simulink model "SWC_CGW_type"  (R2021b)
settings: Solver=FixedStepDiscrete  StartTime=0.0  StopTime=10.0  RelTol=1e-3
(part 1 of 3)
settings Model: DataDictionary=APPTypes.sldd  Creator=FVT23010  LastModifiedBy=FVT23118
settings DataIOCC: SaveFormat=StructureWithTime
settings OptimizationCC: DefaultParameterBehavior=Inlined  EnhancedBackFolding=on  PassReuseOutputArgsAs=Individual arguments  ZeroExternalMemoryAtStartup=off  ZeroInternalMemoryAtStartup=off  OptimizeBlockOrder=speed  DifferentSizesBufferReuse=on  OptimizationCustomize=off  EfficientTunableParamExpr=on
settings DebuggingCC: ParameterTunabilityLossMsg=error
settings HardwareCC: ProdBitPerPointer=32  ProdBitPerSizeT=32  ProdBitPerPtrDiffT=32  ProdLargestAtomicInteger=Long  ProdLargestAtomicFloat=Double  ProdWordSize=32  ProdLongLongMode=on  ProdHWDeviceType=ARM Compatible->ARM Cortex-M
settings ModelReferenceCC: ModelReferenceNumInstancesAllowed=Single
settings SFSimCC: MATLABDynamicMemAlloc=off
settings RTWCC: Description=AUTOSAR  SystemTargetFile=autosar.tlc  GenCodeOnly=on  TemplateMakefile=ert_default_tmf  PortableWordSizes=on
settings CodeAppCC: ForceParamTrailComments=on  IgnoreCustomStorageClasses=off  OperatorAnnotations=on  SimulinkDataObjDesc=on  SFDataObjDesc=on  InsertBlockDesc=on
settings STFCustomTargetCC: TargetLangStandard=C99 (ISO)  MultiwordLength=256  ParMdlRefBuildCompliant=on  CompOptLevelCompliant=on  IncludeMdlTerminateFcn=off  CombineOutputUpdateFcns=on  SuppressErrorStatus=on  ERTCustomFileBanners=on  SupportNonFinite=off  SupportComplex=off  SupportContinuousTime=off  SupportNonInlinedSFcns=off  RemoveResetFunc=on  MATLABClassNameForMDSCustomization=Simulink.SoftwareTarget.ERTCustomization  AutosarCompliant=on  GRTInterface=off  UseToolchainInfoCompliant=on  LookupTableObjectStructAxisOrder=2,1,3,4,...  LUTObjectStructOrderEvenSpacing=Size,Table,Breakpoints  SystemTargetFile=autosar.tlc
settings ERTTargetCC: TargetLangStandard=C99 (ISO)  ConcurrentExecutionCompliant=off  IncludeMdlTerminateFcn=off  SuppressErrorStatus=on  SupportNonFinite=off  SupportComplex=off  ModelStepFunctionPrototypeControlCompliant=off  CPPClassGenCompliant=off  AutosarCompliant=on  LookupTableObjectStructAxisOrder=2,1,3,4,...  LUTObjectStructOrderEvenSpacing=Size,Table,Breakpoints  GenerateASAP2=on  InlinedParameterPlacement=NonHierarchical  ERTCustomFileTemplate=example_file_process.tlc  ConvertIfToSwitch=off  SuppressUnreachableDefaultCases=off  BooleanTrueId=true_MatlabRTW  BooleanFalseId=false_MatlabRTW

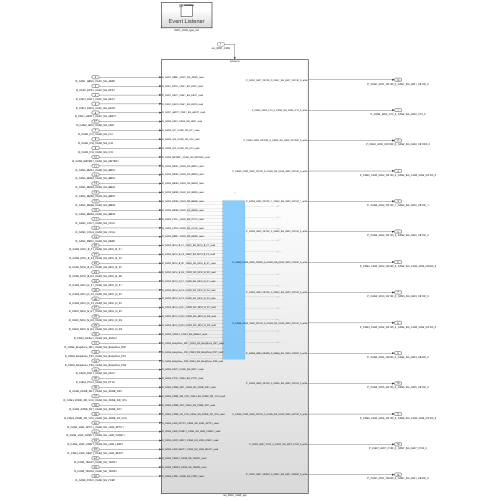
[thumbnail: Simulink's stored preview of the top-level diagram]
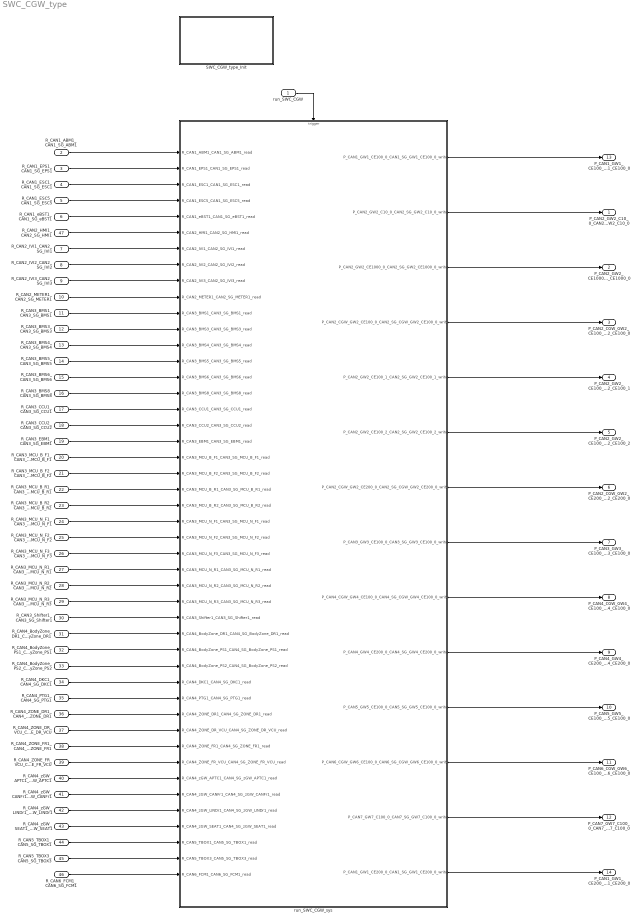
== system SWC_CGW_type ==
  run_SWC_CGW : Inport  OutputFunctionCall=on
  R_CAN1_ABM1_CAN1_SG_ABM1 : Inport  Port=2  OutDataTypeStr=Bus: DT_CAN1_SG_ABM1  PortDimensions=1  BusOutputAsStruct=on
  R_CAN1_EPS1_CAN1_SG_EPS1 : Inport  Port=3  OutDataTypeStr=Bus: DT_CAN1_SG_EPS1  PortDimensions=1  BusOutputAsStruct=on
  R_CAN1_ESC1_CAN1_SG_ESC1 : Inport  Port=4  OutDataTypeStr=Bus: DT_CAN1_SG_ESC1  PortDimensions=1  BusOutputAsStruct=on
  R_CAN1_ESC5_CAN1_SG_ESC5 : Inport  Port=5  OutDataTypeStr=Bus: DT_CAN1_SG_ESC5  PortDimensions=1  BusOutputAsStruct=on
  R_CAN1_eBST1_CAN1_SG_eBST1 : Inport  Port=6  OutDataTypeStr=Bus: DT_CAN1_SG_eBST1  PortDimensions=1  BusOutputAsStruct=on
  R_CAN2_IVI1_CAN2_SG_IVI1 : Inport  Port=7  OutDataTypeStr=Bus: DT_CAN2_SG_IVI1  PortDimensions=1  BusOutputAsStruct=on
  R_CAN2_IVI2_CAN2_SG_IVI2 : Inport  Port=8  OutDataTypeStr=Bus: DT_CAN2_SG_IVI2  PortDimensions=1  BusOutputAsStruct=on
  R_CAN2_IVI3_CAN2_SG_IVI3 : Inport  Port=9  OutDataTypeStr=Bus: DT_CAN2_SG_IVI3  PortDimensions=1  BusOutputAsStruct=on
  R_CAN2_METER1_CAN2_SG_METER1 : Inport  Port=10  OutDataTypeStr=Bus: DT_CAN2_SG_METER1  PortDimensions=1  BusOutputAsStruct=on
  R_CAN3_BMS1_CAN3_SG_BMS1 : Inport  Port=11  OutDataTypeStr=Bus: DT_CAN3_SG_BMS1  PortDimensions=1  BusOutputAsStruct=on
  R_CAN3_BMS3_CAN3_SG_BMS3 : Inport  Port=12  OutDataTypeStr=Bus: DT_CAN3_SG_BMS3  PortDimensions=1  BusOutputAsStruct=on
  R_CAN3_BMS4_CAN3_SG_BMS4 : Inport  Port=13  OutDataTypeStr=Bus: DT_CAN3_SG_BMS4  PortDimensions=1  BusOutputAsStruct=on
  R_CAN3_BMS5_CAN3_SG_BMS5 : Inport  Port=14  OutDataTypeStr=Bus: DT_CAN3_SG_BMS5  PortDimensions=1  BusOutputAsStruct=on
  R_CAN3_BMS6_CAN3_SG_BMS6 : Inport  Port=15  OutDataTypeStr=Bus: DT_CAN3_SG_BMS6  PortDimensions=1  BusOutputAsStruct=on
  R_CAN3_BMS8_CAN3_SG_BMS8 : Inport  Port=16  OutDataTypeStr=Bus: DT_CAN3_SG_BMS8  PortDimensions=1  BusOutputAsStruct=on
  R_CAN3_CCU1_CAN3_SG_CCU1 : Inport  Port=17  OutDataTypeStr=Bus: DT_CAN3_SG_CCU1  PortDimensions=1  BusOutputAsStruct=on
  R_CAN3_CCU2_CAN3_SG_CCU2 : Inport  Port=18  OutDataTypeStr=Bus: DT_CAN3_SG_CCU2  PortDimensions=1  BusOutputAsStruct=on
  R_CAN3_EBM1_CAN3_SG_EBM1 : Inport  Port=19  OutDataTypeStr=Bus: DT_CAN3_SG_EBM1  PortDimensions=1  BusOutputAsStruct=on
  R_CAN3_MCU_B_F1_CAN3_SG_MCU_B_F1 : Inport  Port=20  OutDataTypeStr=Bus: DT_CAN3_SG_MCU_B_F1  PortDimensions=1  BusOutputAsStruct=on
  R_CAN3_MCU_B_F2_CAN3_SG_MCU_B_F2 : Inport  Port=21  OutDataTypeStr=Bus: DT_CAN3_SG_MCU_B_F2  PortDimensions=1  BusOutputAsStruct=on
  R_CAN3_MCU_B_R1_CAN3_SG_MCU_B_R1 : Inport  Port=22  OutDataTypeStr=Bus: DT_CAN3_SG_MCU_B_R1  PortDimensions=1  BusOutputAsStruct=on
  R_CAN3_MCU_B_R2_CAN3_SG_MCU_B_R2 : Inport  Port=23  OutDataTypeStr=Bus: DT_CAN3_SG_MCU_B_R2  PortDimensions=1  BusOutputAsStruct=on
  R_CAN3_MCU_N_F1_CAN3_SG_MCU_N_F1 : Inport  Port=24  OutDataTypeStr=Bus: DT_CAN3_SG_MCU_N_F1  PortDimensions=1  BusOutputAsStruct=on
  R_CAN3_MCU_N_F2_CAN3_SG_MCU_N_F2 : Inport  Port=25  OutDataTypeStr=Bus: DT_CAN3_SG_MCU_N_F2  PortDimensions=1  BusOutputAsStruct=on
  R_CAN3_MCU_N_F3_CAN3_SG_MCU_N_F3 : Inport  Port=26  OutDataTypeStr=Bus: DT_CAN3_SG_MCU_N_F3  PortDimensions=1  BusOutputAsStruct=on
  R_CAN3_MCU_N_R1_CAN3_SG_MCU_N_R1 : Inport  Port=27  OutDataTypeStr=Bus: DT_CAN3_SG_MCU_N_R1  PortDimensions=1  BusOutputAsStruct=on
  R_CAN3_MCU_N_R2_CAN3_SG_MCU_N_R2 : Inport  Port=28  OutDataTypeStr=Bus: DT_CAN3_SG_MCU_N_R2  PortDimensions=1  BusOutputAsStruct=on
  R_CAN3_MCU_N_R3_CAN3_SG_MCU_N_R3 : Inport  Port=29  OutDataTypeStr=Bus: DT_CAN3_SG_MCU_N_R3  PortDimensions=1  BusOutputAsStruct=on
  R_CAN3_Shifter1_CAN3_SG_Shifter1 : Inport  Port=30  OutDataTypeStr=Bus: DT_CAN3_SG_Shifter1  PortDimensions=1  BusOutputAsStruct=on
  R_CAN4_BodyZone_DR1_CAN4_SG_BodyZone_DR1 : Inport  Port=31  OutDataTypeStr=Bus: DT_CAN4_SG_BodyZone_DR1  PortDimensions=1  BusOutputAsStruct=on
  R_CAN4_BodyZone_PS1_CAN4_SG_BodyZone_PS1 : Inport  Port=32  OutDataTypeStr=Bus: DT_CAN4_SG_BodyZone_PS1  PortDimensions=1  BusOutputAsStruct=on
  R_CAN4_BodyZone_PS2_CAN4_SG_BodyZone_PS2 : Inport  Port=33  OutDataTypeStr=Bus: DT_CAN4_SG_BodyZone_PS2  PortDimensions=1  BusOutputAsStruct=on
  R_CAN4_DKC1_CAN4_SG_DKC1 : Inport  Port=34  OutDataTypeStr=Bus: DT_CAN4_SG_DKC1  PortDimensions=1  BusOutputAsStruct=on
  R_CAN4_PTG1_CAN4_SG_PTG1 : Inport  Port=35  OutDataTypeStr=Bus: DT_CAN4_SG_PTG1  PortDimensions=1  BusOutputAsStruct=on
  R_CAN4_ZONE_DR1_CAN4_SG_ZONE_DR1 : Inport  Port=36  OutDataTypeStr=Bus: DT_CAN4_SG_ZONE_DR1  PortDimensions=1  BusOutputAsStruct=on
  R_CAN4_ZONE_DR_VCU_CAN4_SG_ZONE_DR_VCU : Inport  Port=37  OutDataTypeStr=Bus: DT_CAN4_SG_ZONE_DR_VCU  PortDimensions=1  BusOutputAsStruct=on
  R_CAN4_ZONE_FR1_CAN4_SG_ZONE_FR1 : Inport  Port=38  OutDataTypeStr=Bus: DT_CAN4_SG_ZONE_FR1  PortDimensions=1  BusOutputAsStruct=on
  R_CAN4_ZONE_FR_VCU_CAN4_SG_ZONE_FR_VCU : Inport  Port=39  OutDataTypeStr=Bus: DT_CAN4_SG_ZONE_FR_VCU  PortDimensions=1  BusOutputAsStruct=on
  R_CAN4_zGW_APTC1_CAN4_SG_zGW_APTC1 : Inport  Port=40  OutDataTypeStr=Bus: DT_CAN4_SG_zGW_APTC1  PortDimensions=1  BusOutputAsStruct=on
  R_CAN4_zGW_CANFr1_CAN4_SG_zGW_CANFr1 : Inport  Port=41  OutDataTypeStr=Bus: DT_CAN4_SG_zGW_CANFr1  PortDimensions=1  BusOutputAsStruct=on
  R_CAN4_zGW_LINDr1_CAN4_SG_zGW_LINDr1 : Inport  Port=42  OutDataTypeStr=Bus: DT_CAN4_SG_zGW_LINDr1  PortDimensions=1  BusOutputAsStruct=on
  R_CAN4_zGW_SEAT1_CAN4_SG_zGW_SEAT1 : Inport  Port=43  OutDataTypeStr=Bus: DT_CAN4_SG_zGW_SEAT1  PortDimensions=1  BusOutputAsStruct=on
  R_CAN5_TBOX1_CAN5_SG_TBOX1 : Inport  Port=44  OutDataTypeStr=Bus: DT_CAN5_SG_TBOX1  PortDimensions=1  BusOutputAsStruct=on
  R_CAN5_TBOX3_CAN5_SG_TBOX3 : Inport  Port=45  OutDataTypeStr=Bus: DT_CAN5_SG_TBOX3  PortDimensions=1  BusOutputAsStruct=on
  R_CAN6_FCM1_CAN6_SG_FCM1 : Inport  Port=46  OutDataTypeStr=Bus: DT_CAN6_SG_FCM1  PortDimensions=1  BusOutputAsStruct=on
  R_CAN2_HMI1_CAN2_SG_HMI1 : Inport  Port=47  OutDataTypeStr=Bus: DT_CAN2_SG_HMI1  PortDimensions=1  BusOutputAsStruct=on
  SWC_CGW_type_Init : Subsystem
  run_SWC_CGW_sys : Subsystem
  P_CAN2_GW2_C10_0_CAN2_SG_GW2_C10_0 : Outport  OutDataTypeStr=Bus: DT_CAN2_SG_GW2_C10_0  PortDimensions=1  BusOutputAsStruct=on
  P_CAN2_GW2_CE1000_0_CAN2_SG_GW2_CE1000_0 : Outport  Port=2  OutDataTypeStr=Bus: DT_CAN2_SG_GW2_CE1000_0  PortDimensions=1  BusOutputAsStruct=on
  P_CAN2_CGW_GW2_CE100_0_CAN2_SG_CGW_GW2_CE100_0 : Outport  Port=3  OutDataTypeStr=Bus: DT_CAN2_SG_CGW_GW2_CE100_0  PortDimensions=1  BusOutputAsStruct=on
  P_CAN2_GW2_CE100_1_CAN2_SG_GW2_CE100_1 : Outport  Port=4  OutDataTypeStr=Bus: DT_CAN2_SG_GW2_CE100_1  PortDimensions=1  BusOutputAsStruct=on
  P_CAN2_GW2_CE100_2_CAN2_SG_GW2_CE100_2 : Outport  Port=5  OutDataTypeStr=Bus: DT_CAN2_SG_GW2_CE100_2  PortDimensions=1  BusOutputAsStruct=on
  P_CAN2_CGW_GW2_CE200_0_CAN2_SG_CGW_GW2_CE200_0 : Outport  Port=6  OutDataTypeStr=Bus: DT_CAN2_SG_CGW_GW2_CE200_0  PortDimensions=1  BusOutputAsStruct=on
  P_CAN3_GW3_CE100_0_CAN3_SG_GW3_CE100_0 : Outport  Port=7  OutDataTypeStr=Bus: DT_CAN3_SG_GW3_CE100_0  PortDimensions=1  BusOutputAsStruct=on
  P_CAN4_CGW_GW4_CE100_0_CAN4_SG_CGW_GW4_CE100_0 : Outport  Port=8  OutDataTypeStr=Bus: DT_CAN4_SG_CGW_GW4_CE100_0  PortDimensions=1  BusOutputAsStruct=on
  P_CAN4_GW4_CE200_0_CAN4_SG_GW4_CE200_0 : Outport  Port=9  OutDataTypeStr=Bus: DT_CAN4_SG_GW4_CE200_0  PortDimensions=1  BusOutputAsStruct=on
  P_CAN5_GW5_CE100_0_CAN5_SG_GW5_CE100_0 : Outport  Port=10  OutDataTypeStr=Bus: DT_CAN5_SG_GW5_CE100_0  PortDimensions=1  BusOutputAsStruct=on
  P_CAN6_CGW_GW6_CE100_0_CAN6_SG_CGW_GW6_CE100_0 : Outport  Port=11  OutDataTypeStr=Bus: DT_CAN6_SG_CGW_GW6_CE100_0  PortDimensions=1  BusOutputAsStruct=on
  P_CAN7_GW7_C100_0_CAN7_SG_GW7_C100_0 : Outport  Port=12  OutDataTypeStr=Bus: DT_CAN7_SG_GW7_C100_0  PortDimensions=1  BusOutputAsStruct=on
  P_CAN1_GW1_CE100_0_CAN1_SG_GW1_CE100_0 : Outport  Port=13  OutDataTypeStr=Bus: DT_CAN1_SG_GW1_CE100_0  PortDimensions=1  BusOutputAsStruct=on
  P_CAN1_GW1_CE200_0_CAN1_SG_GW1_CE200_0 : Outport  Port=14  OutDataTypeStr=Bus: DT_CAN1_SG_GW1_CE200_0  PortDimensions=1  BusOutputAsStruct=on
  wires:
  R_CAN1_ABM1_CAN1_SG_ABM1/1 -> run_SWC_CGW_sys/1(R_CAN1_ABM1_CAN1_SG_ABM1_read)
  R_CAN1_EPS1_CAN1_SG_EPS1/1 -> run_SWC_CGW_sys/2(R_CAN1_EPS1_CAN1_SG_EPS1_read)
  R_CAN1_ESC1_CAN1_SG_ESC1/1 -> run_SWC_CGW_sys/3(R_CAN1_ESC1_CAN1_SG_ESC1_read)
  R_CAN1_ESC5_CAN1_SG_ESC5/1 -> run_SWC_CGW_sys/4(R_CAN1_ESC5_CAN1_SG_ESC5_read)
  R_CAN1_eBST1_CAN1_SG_eBST1/1 -> run_SWC_CGW_sys/5(R_CAN1_eBST1_CAN1_SG_eBST1_read)
  R_CAN2_IVI1_CAN2_SG_IVI1/1 -> run_SWC_CGW_sys/7(R_CAN2_IVI1_CAN2_SG_IVI1_read)
  R_CAN2_IVI2_CAN2_SG_IVI2/1 -> run_SWC_CGW_sys/8(R_CAN2_IVI2_CAN2_SG_IVI2_read)
  R_CAN2_IVI3_CAN2_SG_IVI3/1 -> run_SWC_CGW_sys/9(R_CAN2_IVI3_CAN2_SG_IVI3_read)
  R_CAN2_METER1_CAN2_SG_METER1/1 -> run_SWC_CGW_sys/10(R_CAN2_METER1_CAN2_SG_METER1_read)
  R_CAN3_BMS1_CAN3_SG_BMS1/1 -> run_SWC_CGW_sys/11(R_CAN3_BMS1_CAN3_SG_BMS1_read)
  R_CAN3_BMS3_CAN3_SG_BMS3/1 -> run_SWC_CGW_sys/12(R_CAN3_BMS3_CAN3_SG_BMS3_read)
  R_CAN3_BMS4_CAN3_SG_BMS4/1 -> run_SWC_CGW_sys/13(R_CAN3_BMS4_CAN3_SG_BMS4_read)
  R_CAN3_BMS5_CAN3_SG_BMS5/1 -> run_SWC_CGW_sys/14(R_CAN3_BMS5_CAN3_SG_BMS5_read)
  R_CAN3_BMS6_CAN3_SG_BMS6/1 -> run_SWC_CGW_sys/15(R_CAN3_BMS6_CAN3_SG_BMS6_read)
  R_CAN3_BMS8_CAN3_SG_BMS8/1 -> run_SWC_CGW_sys/16(R_CAN3_BMS8_CAN3_SG_BMS8_read)
  R_CAN3_CCU1_CAN3_SG_CCU1/1 -> run_SWC_CGW_sys/17(R_CAN3_CCU1_CAN3_SG_CCU1_read)
  R_CAN3_CCU2_CAN3_SG_CCU2/1 -> run_SWC_CGW_sys/18(R_CAN3_CCU2_CAN3_SG_CCU2_read)
  R_CAN3_EBM1_CAN3_SG_EBM1/1 -> run_SWC_CGW_sys/19(R_CAN3_EBM1_CAN3_SG_EBM1_read)
  R_CAN3_MCU_B_F1_CAN3_SG_MCU_B_F1/1 -> run_SWC_CGW_sys/20(R_CAN3_MCU_B_F1_CAN3_SG_MCU_B_F1_read)
  R_CAN3_MCU_B_F2_CAN3_SG_MCU_B_F2/1 -> run_SWC_CGW_sys/21(R_CAN3_MCU_B_F2_CAN3_SG_MCU_B_F2_read)
  R_CAN3_MCU_B_R1_CAN3_SG_MCU_B_R1/1 -> run_SWC_CGW_sys/22(R_CAN3_MCU_B_R1_CAN3_SG_MCU_B_R1_read)
  R_CAN3_MCU_B_R2_CAN3_SG_MCU_B_R2/1 -> run_SWC_CGW_sys/23(R_CAN3_MCU_B_R2_CAN3_SG_MCU_B_R2_read)
  R_CAN3_MCU_N_F1_CAN3_SG_MCU_N_F1/1 -> run_SWC_CGW_sys/24(R_CAN3_MCU_N_F1_CAN3_SG_MCU_N_F1_read)
  R_CAN3_MCU_N_F2_CAN3_SG_MCU_N_F2/1 -> run_SWC_CGW_sys/25(R_CAN3_MCU_N_F2_CAN3_SG_MCU_N_F2_read)
  R_CAN3_MCU_N_F3_CAN3_SG_MCU_N_F3/1 -> run_SWC_CGW_sys/26(R_CAN3_MCU_N_F3_CAN3_SG_MCU_N_F3_read)
  R_CAN3_MCU_N_R1_CAN3_SG_MCU_N_R1/1 -> run_SWC_CGW_sys/27(R_CAN3_MCU_N_R1_CAN3_SG_MCU_N_R1_read)
  R_CAN3_MCU_N_R2_CAN3_SG_MCU_N_R2/1 -> run_SWC_CGW_sys/28(R_CAN3_MCU_N_R2_CAN3_SG_MCU_N_R2_read)
  R_CAN3_MCU_N_R3_CAN3_SG_MCU_N_R3/1 -> run_SWC_CGW_sys/29(R_CAN3_MCU_N_R3_CAN3_SG_MCU_N_R3_read)
  R_CAN3_Shifter1_CAN3_SG_Shifter1/1 -> run_SWC_CGW_sys/30(R_CAN3_Shifter1_CAN3_SG_Shifter1_read)
  R_CAN4_BodyZone_DR1_CAN4_SG_BodyZone_DR1/1 -> run_SWC_CGW_sys/31(R_CAN4_BodyZone_DR1_CAN4_SG_BodyZone_DR1_read)
  R_CAN4_BodyZone_PS1_CAN4_SG_BodyZone_PS1/1 -> run_SWC_CGW_sys/32(R_CAN4_BodyZone_PS1_CAN4_SG_BodyZone_PS1_read)
  R_CAN4_BodyZone_PS2_CAN4_SG_BodyZone_PS2/1 -> run_SWC_CGW_sys/33(R_CAN4_BodyZone_PS2_CAN4_SG_BodyZone_PS2_read)
  R_CAN4_DKC1_CAN4_SG_DKC1/1 -> run_SWC_CGW_sys/34(R_CAN4_DKC1_CAN4_SG_DKC1_read)
  R_CAN4_PTG1_CAN4_SG_PTG1/1 -> run_SWC_CGW_sys/35(R_CAN4_PTG1_CAN4_SG_PTG1_read)
  R_CAN4_ZONE_DR1_CAN4_SG_ZONE_DR1/1 -> run_SWC_CGW_sys/36(R_CAN4_ZONE_DR1_CAN4_SG_ZONE_DR1_read)
  R_CAN4_ZONE_DR_VCU_CAN4_SG_ZONE_DR_VCU/1 -> run_SWC_CGW_sys/37(R_CAN4_ZONE_DR_VCU_CAN4_SG_ZONE_DR_VCU_read)
  R_CAN4_ZONE_FR1_CAN4_SG_ZONE_FR1/1 -> run_SWC_CGW_sys/38(R_CAN4_ZONE_FR1_CAN4_SG_ZONE_FR1_read)
  R_CAN4_ZONE_FR_VCU_CAN4_SG_ZONE_FR_VCU/1 -> run_SWC_CGW_sys/39(R_CAN4_ZONE_FR_VCU_CAN4_SG_ZONE_FR_VCU_read)
  R_CAN4_zGW_APTC1_CAN4_SG_zGW_APTC1/1 -> run_SWC_CGW_sys/40(R_CAN4_zGW_APTC1_CAN4_SG_zGW_APTC1_read)
  R_CAN4_zGW_CANFr1_CAN4_SG_zGW_CANFr1/1 -> run_SWC_CGW_sys/41(R_CAN4_zGW_CANFr1_CAN4_SG_zGW_CANFr1_read)
  R_CAN4_zGW_LINDr1_CAN4_SG_zGW_LINDr1/1 -> run_SWC_CGW_sys/42(R_CAN4_zGW_LINDr1_CAN4_SG_zGW_LINDr1_read)
  R_CAN4_zGW_SEAT1_CAN4_SG_zGW_SEAT1/1 -> run_SWC_CGW_sys/43(R_CAN4_zGW_SEAT1_CAN4_SG_zGW_SEAT1_read)
  R_CAN5_TBOX1_CAN5_SG_TBOX1/1 -> run_SWC_CGW_sys/44(R_CAN5_TBOX1_CAN5_SG_TBOX1_read)
  R_CAN5_TBOX3_CAN5_SG_TBOX3/1 -> run_SWC_CGW_sys/45(R_CAN5_TBOX3_CAN5_SG_TBOX3_read)
  R_CAN6_FCM1_CAN6_SG_FCM1/1 -> run_SWC_CGW_sys/46(R_CAN6_FCM1_CAN6_SG_FCM1_read)
  run_SWC_CGW/1 -> run_SWC_CGW_sys/Trigger
  R_CAN2_HMI1_CAN2_SG_HMI1/1 -> run_SWC_CGW_sys/6(R_CAN2_HMI1_CAN2_SG_HMI1_read)
  run_SWC_CGW_sys/2(P_CAN2_GW2_C10_0_CAN2_SG_GW2_C10_0_write) -> P_CAN2_GW2_C10_0_CAN2_SG_GW2_C10_0/1
  run_SWC_CGW_sys/3(P_CAN2_GW2_CE1000_0_CAN2_SG_GW2_CE1000_0_write) -> P_CAN2_GW2_CE1000_0_CAN2_SG_GW2_CE1000_0/1
  run_SWC_CGW_sys/4(P_CAN2_CGW_GW2_CE100_0_CAN2_SG_CGW_GW2_CE100_0_write) -> P_CAN2_CGW_GW2_CE100_0_CAN2_SG_CGW_GW2_CE100_0/1
  run_SWC_CGW_sys/5(P_CAN2_GW2_CE100_1_CAN2_SG_GW2_CE100_1_write) -> P_CAN2_GW2_CE100_1_CAN2_SG_GW2_CE100_1/1
  run_SWC_CGW_sys/6(P_CAN2_GW2_CE100_2_CAN2_SG_GW2_CE100_2_write) -> P_CAN2_GW2_CE100_2_CAN2_SG_GW2_CE100_2/1
  run_SWC_CGW_sys/7(P_CAN2_CGW_GW2_CE200_0_CAN2_SG_CGW_GW2_CE200_0_write) -> P_CAN2_CGW_GW2_CE200_0_CAN2_SG_CGW_GW2_CE200_0/1
  run_SWC_CGW_sys/8(P_CAN3_GW3_CE100_0_CAN3_SG_GW3_CE100_0_write) -> P_CAN3_GW3_CE100_0_CAN3_SG_GW3_CE100_0/1
  run_SWC_CGW_sys/9(P_CAN4_CGW_GW4_CE100_0_CAN4_SG_CGW_GW4_CE100_0_write) -> P_CAN4_CGW_GW4_CE100_0_CAN4_SG_CGW_GW4_CE100_0/1
  run_SWC_CGW_sys/10(P_CAN4_GW4_CE200_0_CAN4_SG_GW4_CE200_0_write) -> P_CAN4_GW4_CE200_0_CAN4_SG_GW4_CE200_0/1
  run_SWC_CGW_sys/11(P_CAN5_GW5_CE100_0_CAN5_SG_GW5_CE100_0_write) -> P_CAN5_GW5_CE100_0_CAN5_SG_GW5_CE100_0/1
  run_SWC_CGW_sys/12(P_CAN6_CGW_GW6_CE100_0_CAN6_SG_CGW_GW6_CE100_0_write) -> P_CAN6_CGW_GW6_CE100_0_CAN6_SG_CGW_GW6_CE100_0/1
  run_SWC_CGW_sys/1(P_CAN1_GW1_CE100_0_CAN1_SG_GW1_CE100_0_write) -> P_CAN1_GW1_CE100_0_CAN1_SG_GW1_CE100_0/1
  run_SWC_CGW_sys/13(P_CAN7_GW7_C100_0_CAN7_SG_GW7_C100_0_write) -> P_CAN7_GW7_C100_0_CAN7_SG_GW7_C100_0/1
  run_SWC_CGW_sys/14(P_CAN1_GW1_CE200_0_CAN1_SG_GW1_CE200_0_write) -> P_CAN1_GW1_CE200_0_CAN1_SG_GW1_CE200_0/1

== system SWC_CGW_type/SWC_CGW_type_Init ==
  Event Listener : EventListener  EventName=reset

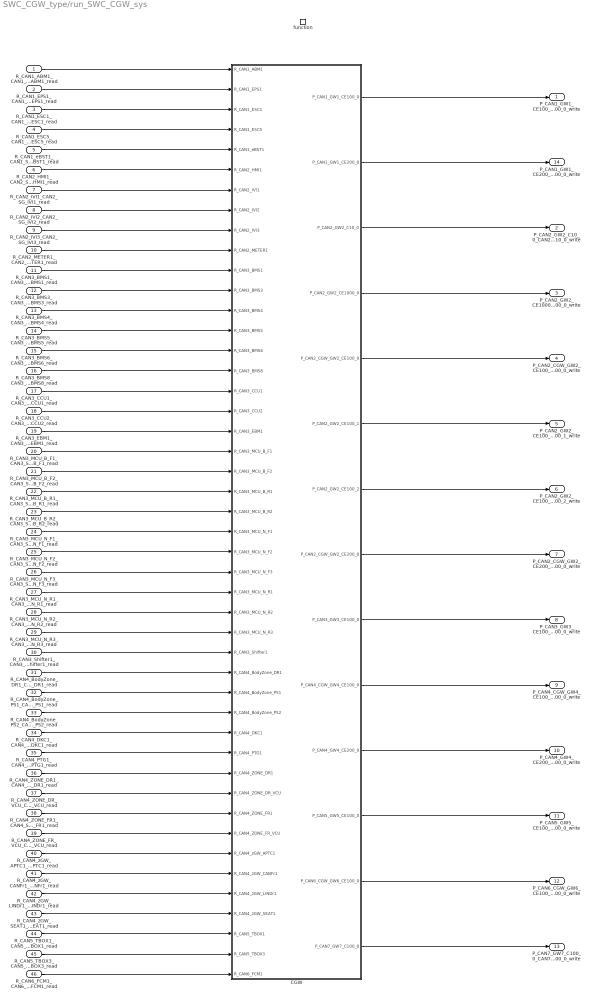
== system SWC_CGW_type/run_SWC_CGW_sys ==
  R_CAN1_ABM1_CAN1_SG_ABM1_read : Inport
  R_CAN1_EPS1_CAN1_SG_EPS1_read : Inport  Port=2
  R_CAN1_ESC1_CAN1_SG_ESC1_read : Inport  Port=3
  R_CAN1_ESC5_CAN1_SG_ESC5_read : Inport  Port=4
  R_CAN1_eBST1_CAN1_SG_eBST1_read : Inport  Port=5
  R_CAN2_HMI1_CAN2_SG_HMI1_read : Inport  Port=6
  R_CAN2_IVI1_CAN2_SG_IVI1_read : Inport  Port=7
  R_CAN2_IVI2_CAN2_SG_IVI2_read : Inport  Port=8
  R_CAN2_IVI3_CAN2_SG_IVI3_read : Inport  Port=9
  R_CAN2_METER1_CAN2_SG_METER1_read : Inport  Port=10
  R_CAN3_BMS1_CAN3_SG_BMS1_read : Inport  Port=11
  R_CAN3_BMS3_CAN3_SG_BMS3_read : Inport  Port=12
  R_CAN3_BMS4_CAN3_SG_BMS4_read : Inport  Port=13
  R_CAN3_BMS5_CAN3_SG_BMS5_read : Inport  Port=14
  R_CAN3_BMS6_CAN3_SG_BMS6_read : Inport  Port=15
  R_CAN3_BMS8_CAN3_SG_BMS8_read : Inport  Port=16
  R_CAN3_CCU1_CAN3_SG_CCU1_read : Inport  Port=17
  R_CAN3_CCU2_CAN3_SG_CCU2_read : Inport  Port=18
  R_CAN3_EBM1_CAN3_SG_EBM1_read : Inport  Port=19
  R_CAN3_MCU_B_F1_CAN3_SG_MCU_B_F1_read : Inport  Port=20
  R_CAN3_MCU_B_F2_CAN3_SG_MCU_B_F2_read : Inport  Port=21
  R_CAN3_MCU_B_R1_CAN3_SG_MCU_B_R1_read : Inport  Port=22
  R_CAN3_MCU_B_R2_CAN3_SG_MCU_B_R2_read : Inport  Port=23
  R_CAN3_MCU_N_F1_CAN3_SG_MCU_N_F1_read : Inport  Port=24
  R_CAN3_MCU_N_F2_CAN3_SG_MCU_N_F2_read : Inport  Port=25
  R_CAN3_MCU_N_F3_CAN3_SG_MCU_N_F3_read : Inport  Port=26
  R_CAN3_MCU_N_R1_CAN3_SG_MCU_N_R1_read : Inport  Port=27
  R_CAN3_MCU_N_R2_CAN3_SG_MCU_N_R2_read : Inport  Port=28
  R_CAN3_MCU_N_R3_CAN3_SG_MCU_N_R3_read : Inport  Port=29
  R_CAN3_Shifter1_CAN3_SG_Shifter1_read : Inport  Port=30
  R_CAN4_BodyZone_DR1_CAN4_SG_BodyZone_DR1_read : Inport  Port=31
  R_CAN4_BodyZone_PS1_CAN4_SG_BodyZone_PS1_read : Inport  Port=32
  R_CAN4_BodyZone_PS2_CAN4_SG_BodyZone_PS2_read : Inport  Port=33
  R_CAN4_DKC1_CAN4_SG_DKC1_read : Inport  Port=34
  R_CAN4_PTG1_CAN4_SG_PTG1_read : Inport  Port=35
  R_CAN4_ZONE_DR1_CAN4_SG_ZONE_DR1_read : Inport  Port=36
  R_CAN4_ZONE_DR_VCU_CAN4_SG_ZONE_DR_VCU_read : Inport  Port=37
  R_CAN4_ZONE_FR1_CAN4_SG_ZONE_FR1_read : Inport  Port=38
  R_CAN4_ZONE_FR_VCU_CAN4_SG_ZONE_FR_VCU_read : Inport  Port=39
  R_CAN4_zGW_APTC1_CAN4_SG_zGW_APTC1_read : Inport  Port=40
  R_CAN4_zGW_CANFr1_CAN4_SG_zGW_CANFr1_read : Inport  Port=41
  R_CAN4_zGW_LINDr1_CAN4_SG_zGW_LINDr1_read : Inport  Port=42
  R_CAN4_zGW_SEAT1_CAN4_SG_zGW_SEAT1_read : Inport  Port=43
  R_CAN5_TBOX1_CAN5_SG_TBOX1_read : Inport  Port=44
  R_CAN5_TBOX3_CAN5_SG_TBOX3_read : Inport  Port=45
  R_CAN6_FCM1_CAN6_SG_FCM1_read : Inport  Port=46
  function : TriggerPort  TriggerType=function-call  VariantControl=(inherit)
  CGW : Subsystem
  P_CAN1_GW1_CE100_0_CAN1_SG_GW1_CE100_0_write : Outport
  P_CAN2_GW2_C10_0_CAN2_SG_GW2_C10_0_write : Outport  Port=2
  P_CAN2_GW2_CE1000_0_CAN2_SG_GW2_CE1000_0_write : Outport  Port=3
  P_CAN2_CGW_GW2_CE100_0_CAN2_SG_CGW_GW2_CE100_0_write : Outport  Port=4
  P_CAN2_GW2_CE100_1_CAN2_SG_GW2_CE100_1_write : Outport  Port=5
  P_CAN2_GW2_CE100_2_CAN2_SG_GW2_CE100_2_write : Outport  Port=6
  P_CAN2_CGW_GW2_CE200_0_CAN2_SG_CGW_GW2_CE200_0_write : Outport  Port=7
  P_CAN3_GW3_CE100_0_CAN3_SG_GW3_CE100_0_write : Outport  Port=8
  P_CAN4_CGW_GW4_CE100_0_CAN4_SG_CGW_GW4_CE100_0_write : Outport  Port=9
  P_CAN4_GW4_CE200_0_CAN4_SG_GW4_CE200_0_write : Outport  Port=10
  P_CAN5_GW5_CE100_0_CAN5_SG_GW5_CE100_0_write : Outport  Port=11
  P_CAN6_CGW_GW6_CE100_0_CAN6_SG_CGW_GW6_CE100_0_write : Outport  Port=12
  P_CAN7_GW7_C100_0_CAN7_SG_GW7_C100_0_write : Outport  Port=13
  P_CAN1_GW1_CE200_0_CAN1_SG_GW1_CE200_0_write : Outport  Port=14
  wires:
  R_CAN1_ABM1_CAN1_SG_ABM1_read/1 -> CGW/1(R_CAN1_ABM1)
  R_CAN1_EPS1_CAN1_SG_EPS1_read/1 -> CGW/2(R_CAN1_EPS1)
  R_CAN1_ESC1_CAN1_SG_ESC1_read/1 -> CGW/3(R_CAN1_ESC1)
  R_CAN1_ESC5_CAN1_SG_ESC5_read/1 -> CGW/4(R_CAN1_ESC5)
  R_CAN1_eBST1_CAN1_SG_eBST1_read/1 -> CGW/5(R_CAN1_eBST1)
  R_CAN2_HMI1_CAN2_SG_HMI1_read/1 -> CGW/6(R_CAN2_HMI1)
  R_CAN2_IVI1_CAN2_SG_IVI1_read/1 -> CGW/7(R_CAN2_IVI1)
  R_CAN2_IVI2_CAN2_SG_IVI2_read/1 -> CGW/8(R_CAN2_IVI2)
  R_CAN2_IVI3_CAN2_SG_IVI3_read/1 -> CGW/9(R_CAN2_IVI3)
  R_CAN2_METER1_CAN2_SG_METER1_read/1 -> CGW/10(R_CAN2_METER1)
  R_CAN3_BMS1_CAN3_SG_BMS1_read/1 -> CGW/11(R_CAN3_BMS1)
  R_CAN3_BMS3_CAN3_SG_BMS3_read/1 -> CGW/12(R_CAN3_BMS3)
  R_CAN3_BMS4_CAN3_SG_BMS4_read/1 -> CGW/13(R_CAN3_BMS4)
  R_CAN3_BMS5_CAN3_SG_BMS5_read/1 -> CGW/14(R_CAN3_BMS5)
  R_CAN3_BMS6_CAN3_SG_BMS6_read/1 -> CGW/15(R_CAN3_BMS6)
  R_CAN3_BMS8_CAN3_SG_BMS8_read/1 -> CGW/16(R_CAN3_BMS8)
  R_CAN3_CCU1_CAN3_SG_CCU1_read/1 -> CGW/17(R_CAN3_CCU1)
  R_CAN3_CCU2_CAN3_SG_CCU2_read/1 -> CGW/18(R_CAN3_CCU2)
  R_CAN3_EBM1_CAN3_SG_EBM1_read/1 -> CGW/19(R_CAN3_EBM1)
  R_CAN3_MCU_B_F1_CAN3_SG_MCU_B_F1_read/1 -> CGW/20(R_CAN3_MCU_B_F1)
  R_CAN3_MCU_B_F2_CAN3_SG_MCU_B_F2_read/1 -> CGW/21(R_CAN3_MCU_B_F2)
  R_CAN3_MCU_B_R1_CAN3_SG_MCU_B_R1_read/1 -> CGW/22(R_CAN3_MCU_B_R1)
  R_CAN3_MCU_B_R2_CAN3_SG_MCU_B_R2_read/1 -> CGW/23(R_CAN3_MCU_B_R2)
  R_CAN3_MCU_N_F1_CAN3_SG_MCU_N_F1_read/1 -> CGW/24(R_CAN3_MCU_N_F1)
  R_CAN3_MCU_N_F2_CAN3_SG_MCU_N_F2_read/1 -> CGW/25(R_CAN3_MCU_N_F2)
  R_CAN3_MCU_N_F3_CAN3_SG_MCU_N_F3_read/1 -> CGW/26(R_CAN3_MCU_N_F3)
  R_CAN3_MCU_N_R1_CAN3_SG_MCU_N_R1_read/1 -> CGW/27(R_CAN3_MCU_N_R1)
  R_CAN3_MCU_N_R2_CAN3_SG_MCU_N_R2_read/1 -> CGW/28(R_CAN3_MCU_N_R2)
  R_CAN3_MCU_N_R3_CAN3_SG_MCU_N_R3_read/1 -> CGW/29(R_CAN3_MCU_N_R3)
  R_CAN3_Shifter1_CAN3_SG_Shifter1_read/1 -> CGW/30(R_CAN3_Shifter1)
  R_CAN4_BodyZone_DR1_CAN4_SG_BodyZone_DR1_read/1 -> CGW/31(R_CAN4_BodyZone_DR1)
  CGW/1(P_CAN1_GW1_CE100_0) -> P_CAN1_GW1_CE100_0_CAN1_SG_GW1_CE100_0_write/1
  CGW/2(P_CAN1_GW1_CE200_0) -> P_CAN1_GW1_CE200_0_CAN1_SG_GW1_CE200_0_write/1
  CGW/3(P_CAN2_GW2_C10_0) -> P_CAN2_GW2_C10_0_CAN2_SG_GW2_C10_0_write/1
  CGW/4(P_CAN2_GW2_CE1000_0) -> P_CAN2_GW2_CE1000_0_CAN2_SG_GW2_CE1000_0_write/1
  CGW/5(P_CAN2_CGW_GW2_CE100_0) -> P_CAN2_CGW_GW2_CE100_0_CAN2_SG_CGW_GW2_CE100_0_write/1
  CGW/6(P_CAN2_GW2_CE100_1) -> P_CAN2_GW2_CE100_1_CAN2_SG_GW2_CE100_1_write/1
  CGW/7(P_CAN2_GW2_CE100_2) -> P_CAN2_GW2_CE100_2_CAN2_SG_GW2_CE100_2_write/1
  CGW/8(P_CAN2_CGW_GW2_CE200_0) -> P_CAN2_CGW_GW2_CE200_0_CAN2_SG_CGW_GW2_CE200_0_write/1
  CGW/9(P_CAN3_GW3_CE100_0) -> P_CAN3_GW3_CE100_0_CAN3_SG_GW3_CE100_0_write/1
  CGW/10(P_CAN4_CGW_GW4_CE100_0) -> P_CAN4_CGW_GW4_CE100_0_CAN4_SG_CGW_GW4_CE100_0_write/1
  CGW/11(P_CAN4_GW4_CE200_0) -> P_CAN4_GW4_CE200_0_CAN4_SG_GW4_CE200_0_write/1
  CGW/12(P_CAN5_GW5_CE100_0) -> P_CAN5_GW5_CE100_0_CAN5_SG_GW5_CE100_0_write/1
  CGW/13(P_CAN6_CGW_GW6_CE100_0) -> P_CAN6_CGW_GW6_CE100_0_CAN6_SG_CGW_GW6_CE100_0_write/1
  CGW/14(P_CAN7_GW7_C100_0) -> P_CAN7_GW7_C100_0_CAN7_SG_GW7_C100_0_write/1
  R_CAN4_BodyZone_PS1_CAN4_SG_BodyZone_PS1_read/1 -> CGW/32(R_CAN4_BodyZone_PS1)
  R_CAN4_BodyZone_PS2_CAN4_SG_BodyZone_PS2_read/1 -> CGW/33(R_CAN4_BodyZone_PS2)
  R_CAN4_DKC1_CAN4_SG_DKC1_read/1 -> CGW/34(R_CAN4_DKC1)
  R_CAN4_PTG1_CAN4_SG_PTG1_read/1 -> CGW/35(R_CAN4_PTG1)
  R_CAN4_ZONE_DR1_CAN4_SG_ZONE_DR1_read/1 -> CGW/36(R_CAN4_ZONE_DR1)
  R_CAN4_ZONE_DR_VCU_CAN4_SG_ZONE_DR_VCU_read/1 -> CGW/37(R_CAN4_ZONE_DR_VCU)
  R_CAN4_ZONE_FR1_CAN4_SG_ZONE_FR1_read/1 -> CGW/38(R_CAN4_ZONE_FR1)
  R_CAN4_ZONE_FR_VCU_CAN4_SG_ZONE_FR_VCU_read/1 -> CGW/39(R_CAN4_ZONE_FR_VCU)
  R_CAN4_zGW_APTC1_CAN4_SG_zGW_APTC1_read/1 -> CGW/40(R_CAN4_zGW_APTC1)
  R_CAN4_zGW_CANFr1_CAN4_SG_zGW_CANFr1_read/1 -> CGW/41(R_CAN4_zGW_CANFr1)
  R_CAN4_zGW_LINDr1_CAN4_SG_zGW_LINDr1_read/1 -> CGW/42(R_CAN4_zGW_LINDr1)
  R_CAN4_zGW_SEAT1_CAN4_SG_zGW_SEAT1_read/1 -> CGW/43(R_CAN4_zGW_SEAT1)
  R_CAN5_TBOX1_CAN5_SG_TBOX1_read/1 -> CGW/44(R_CAN5_TBOX1)
  R_CAN5_TBOX3_CAN5_SG_TBOX3_read/1 -> CGW/45(R_CAN5_TBOX3)
  R_CAN6_FCM1_CAN6_SG_FCM1_read/1 -> CGW/46(R_CAN6_FCM1)

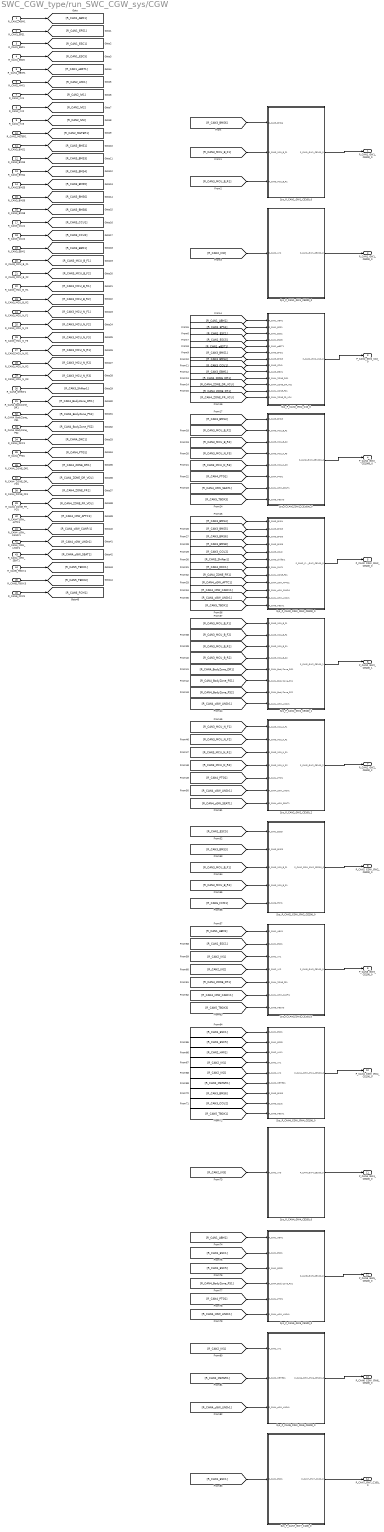
== system SWC_CGW_type/run_SWC_CGW_sys/CGW ==
  R_CAN1_ABM1 : Inport
  R_CAN1_EPS1 : Inport  Port=2
  R_CAN1_ESC1 : Inport  Port=3
  R_CAN1_ESC5 : Inport  Port=4
  R_CAN1_eBST1 : Inport  Port=5
  R_CAN2_HMI1 : Inport  Port=6
  R_CAN2_IVI1 : Inport  Port=7
  R_CAN2_IVI2 : Inport  Port=8
  R_CAN2_IVI3 : Inport  Port=9
  R_CAN2_METER1 : Inport  Port=10
  R_CAN3_BMS1 : Inport  Port=11
  R_CAN3_BMS3 : Inport  Port=12
  R_CAN3_BMS4 : Inport  Port=13
  R_CAN3_BMS5 : Inport  Port=14
  R_CAN3_BMS6 : Inport  Port=15
  R_CAN3_BMS8 : Inport  Port=16
  R_CAN3_CCU1 : Inport  Port=17
  R_CAN3_CCU2 : Inport  Port=18
  R_CAN3_EBM1 : Inport  Port=19
  R_CAN3_MCU_B_F1 : Inport  Port=20
  R_CAN3_MCU_B_F2 : Inport  Port=21
  R_CAN3_MCU_B_R1 : Inport  Port=22
  R_CAN3_MCU_B_R2 : Inport  Port=23
  R_CAN3_MCU_N_F1 : Inport  Port=24
  R_CAN3_MCU_N_F2 : Inport  Port=25
  R_CAN3_MCU_N_F3 : Inport  Port=26
  R_CAN3_MCU_N_R1 : Inport  Port=27
  R_CAN3_MCU_N_R2 : Inport  Port=28
  R_CAN3_MCU_N_R3 : Inport  Port=29
  R_CAN3_Shifter1 : Inport  Port=30
  R_CAN4_BodyZone_DR1 : Inport  Port=31
  R_CAN4_BodyZone_PS1 : Inport  Port=32
  R_CAN4_BodyZone_PS2 : Inport  Port=33
  R_CAN4_DKC1 : Inport  Port=34
  R_CAN4_PTG1 : Inport  Port=35
  R_CAN4_ZONE_DR1 : Inport  Port=36
  R_CAN4_ZONE_DR_VCU : Inport  Port=37
  R_CAN4_ZONE_FR1 : Inport  Port=38
  R_CAN4_ZONE_FR_VCU : Inport  Port=39
  R_CAN4_zGW_APTC1 : Inport  Port=40
  R_CAN4_zGW_CANFr1 : Inport  Port=41
  R_CAN4_zGW_LINDr1 : Inport  Port=42
  R_CAN4_zGW_SEAT1 : Inport  Port=43
  R_CAN5_TBOX1 : Inport  Port=44
  R_CAN5_TBOX3 : Inport  Port=45
  R_CAN6_FCM1 : Inport  Port=46
  Sys_P_CAN1_GW1_CE100_0 : Subsystem
  Sys_P_CAN1_GW1_CE200_0 : Subsystem
  Sys_P_CAN2_CGW_GW2_CE100_0 : Subsystem
  Sys_P_CAN2_CGW_GW2_CE200_0 : Subsystem
  Sys_P_CAN2_GW2_C10_0 : Subsystem
  Sys_P_CAN2_GW2_CE1000_0 : Subsystem
  Sys_P_CAN2_GW2_CE100_1 : Subsystem
  Sys_P_CAN2_GW2_CE100_2 : Subsystem
  Sys_P_CAN3_GW3_CE100_0 : Subsystem
  Sys_P_CAN4_CGW_GW4_CE100_0 : Subsystem
  Sys_P_CAN4_GW4_CE200_0 : Subsystem
  Sys_P_CAN5_GW5_CE100_0 : Subsystem
  Sys_P_CAN6_CGW_GW6_CE100_0 : Subsystem
  Sys_P_CAN7_GW7_C100_0 : Subsystem
  P_CAN1_GW1_CE100_0 : Outport
  P_CAN1_GW1_CE200_0 : Outport  Port=2
  P_CAN2_GW2_C10_0 : Outport  Port=3
  P_CAN2_GW2_CE1000_0 : Outport  Port=4
  P_CAN2_CGW_GW2_CE100_0 : Outport  Port=5
  P_CAN2_GW2_CE100_1 : Outport  Port=6
  P_CAN2_GW2_CE100_2 : Outport  Port=7
  P_CAN2_CGW_GW2_CE200_0 : Outport  Port=8
  P_CAN3_GW3_CE100_0 : Outport  Port=9
  P_CAN4_CGW_GW4_CE100_0 : Outport  Port=10
  P_CAN4_GW4_CE200_0 : Outport  Port=11
  P_CAN5_GW5_CE100_0 : Outport  Port=12
  P_CAN6_CGW_GW6_CE100_0 : Outport  Port=13
  P_CAN7_GW7_C100_0 : Outport  Port=14
  wires:
  R_CAN1_ABM1/1 -> [R_CAN1_ABM1]
  R_CAN1_EPS1/1 -> [R_CAN1_EPS1]
  R_CAN1_ESC1/1 -> [R_CAN1_ESC1]
  R_CAN1_ESC5/1 -> [R_CAN1_ESC5]
  R_CAN1_eBST1/1 -> [R_CAN1_eBST1]
  R_CAN2_HMI1/1 -> [R_CAN2_HMI1]
  R_CAN2_IVI1/1 -> [R_CAN2_IVI1]
  R_CAN2_IVI2/1 -> [R_CAN2_IVI2]
  R_CAN2_IVI3/1 -> [R_CAN2_IVI3]
  R_CAN2_METER1/1 -> [R_CAN2_METER1]
  R_CAN3_BMS1/1 -> [R_CAN3_BMS1]
  R_CAN3_BMS3/1 -> [R_CAN3_BMS3]
  R_CAN3_BMS4/1 -> [R_CAN3_BMS4]
  R_CAN3_BMS5/1 -> [R_CAN3_BMS5]
  R_CAN3_BMS6/1 -> [R_CAN3_BMS6]
  R_CAN3_BMS8/1 -> [R_CAN3_BMS8]
  R_CAN3_CCU1/1 -> [R_CAN3_CCU1]
  R_CAN3_CCU2/1 -> [R_CAN3_CCU2]
  R_CAN3_EBM1/1 -> [R_CAN3_EBM1]
  R_CAN3_MCU_B_F1/1 -> [R_CAN3_MCU_B_F1]
  R_CAN3_MCU_B_F2/1 -> [R_CAN3_MCU_B_F2]
  R_CAN3_MCU_B_R1/1 -> [R_CAN3_MCU_B_R1]
  R_CAN3_MCU_B_R2/1 -> [R_CAN3_MCU_B_R2]
  R_CAN3_MCU_N_F1/1 -> [R_CAN3_MCU_N_F1]
  R_CAN3_MCU_N_F2/1 -> [R_CAN3_MCU_N_F2]
  R_CAN3_MCU_N_F3/1 -> [R_CAN3_MCU_N_F3]
  R_CAN3_MCU_N_R1/1 -> [R_CAN3_MCU_N_R1]
  R_CAN3_MCU_N_R2/1 -> [R_CAN3_MCU_N_R2]
  R_CAN3_MCU_N_R3/1 -> [R_CAN3_MCU_N_R3]
  R_CAN3_Shifter1/1 -> [R_CAN3_Shifter1]
  R_CAN4_BodyZone_DR1/1 -> [R_CAN4_BodyZone_DR1]
  R_CAN4_BodyZone_PS1/1 -> [R_CAN4_BodyZone_PS1]
  R_CAN4_BodyZone_PS2/1 -> [R_CAN4_BodyZone_PS2]
  R_CAN4_DKC1/1 -> [R_CAN4_DKC1]
  R_CAN4_PTG1/1 -> [R_CAN4_PTG1]
  R_CAN4_ZONE_DR1/1 -> [R_CAN4_ZONE_DR1]
  R_CAN4_ZONE_DR_VCU/1 -> [R_CAN4_ZONE_DR_VCU]
  R_CAN4_ZONE_FR1/1 -> [R_CAN4_ZONE_FR1]
  R_CAN4_ZONE_FR_VCU/1 -> [R_CAN4_ZONE_FR_VCU]
  R_CAN4_zGW_APTC1/1 -> [R_CAN4_zGW_APTC1]
  R_CAN4_zGW_CANFr1/1 -> [R_CAN4_zGW_CANFr1]
  R_CAN4_zGW_LINDr1/1 -> [R_CAN4_zGW_LINDr1]
  R_CAN4_zGW_SEAT1/1 -> [R_CAN4_zGW_SEAT1]
  R_CAN5_TBOX1/1 -> [R_CAN5_TBOX1]
  R_CAN5_TBOX3/1 -> [R_CAN5_TBOX3]
  R_CAN6_FCM1/1 -> [R_CAN6_FCM1]
  Sys_P_CAN1_GW1_CE100_0/1(P_CAN1_GW1_CE100_0) -> P_CAN1_GW1_CE100_0/1
  Sys_P_CAN1_GW1_CE200_0/1(P_CAN1_GW1_CE200_0) -> P_CAN1_GW1_CE200_0/1
  Sys_P_CAN2_GW2_C10_0/1(P_CAN2_GW2_C10_0) -> P_CAN2_GW2_C10_0/1
  Sys_P_CAN2_GW2_CE1000_0/1(P_CAN2_GW2_CE1000_0) -> P_CAN2_GW2_CE1000_0/1
  Sys_P_CAN2_CGW_GW2_CE100_0/1(P_CAN2_CGW_GW2_CE100_0) -> P_CAN2_CGW_GW2_CE100_0/1
  Sys_P_CAN2_GW2_CE100_1/1(P_CAN2_GW2_CE100_1) -> P_CAN2_GW2_CE100_1/1
  Sys_P_CAN2_GW2_CE100_2/1(P_CAN2_GW2_CE100_2) -> P_CAN2_GW2_CE100_2/1
  Sys_P_CAN2_CGW_GW2_CE200_0/1(P_CAN2_CGW_GW2_CE200_0) -> P_CAN2_CGW_GW2_CE200_0/1
  Sys_P_CAN3_GW3_CE100_0/1(P_CAN3_GW3_CE100_0) -> P_CAN3_GW3_CE100_0/1
  Sys_P_CAN4_CGW_GW4_CE100_0/1(P_CAN4_CGW_GW4_CE100_0) -> P_CAN4_CGW_GW4_CE100_0/1
  Sys_P_CAN4_GW4_CE200_0/1(P_CAN4_GW4_CE200_0) -> P_CAN4_GW4_CE200_0/1
  Sys_P_CAN5_GW5_CE100_0/1(P_CAN5_GW5_CE100_0) -> P_CAN5_GW5_CE100_0/1
  Sys_P_CAN6_CGW_GW6_CE100_0/1(P_CAN6_CGW_GW6_CE100_0) -> P_CAN6_CGW_GW6_CE100_0/1
  Sys_P_CAN7_GW7_C100_0/1(P_CAN7_GW7_C100_0) -> P_CAN7_GW7_C100_0/1
  [R_CAN3_BMS6] -> Sys_P_CAN1_GW1_CE100_0/1(R_CAN3_BMS6)
  [R_CAN3_MCU_B_F1] -> Sys_P_CAN1_GW1_CE100_0/2(R_CAN3_MCU_B_F1)
  [R_CAN3_MCU_B_R1] -> Sys_P_CAN1_GW1_CE100_0/3(R_CAN3_MCU_B_R1)
  [R_CAN2_IVI2] -> Sys_P_CAN1_GW1_CE200_0/1(R_CAN2_IVI2)
  [R_CAN1_ABM1] -> Sys_P_CAN2_GW2_C10_0/1(R_CAN1_ABM1)
  [R_CAN1_EPS1] -> Sys_P_CAN2_GW2_C10_0/2(R_CAN1_EPS1)
  [R_CAN1_ESC1] -> Sys_P_CAN2_GW2_C10_0/3(R_CAN1_ESC1)
  [R_CAN1_ESC5] -> Sys_P_CAN2_GW2_C10_0/4(R_CAN1_ESC5)
  [R_CAN1_eBST1] -> Sys_P_CAN2_GW2_C10_0/5(R_CAN1_eBST1)
  [R_CAN3_BMS1] -> Sys_P_CAN2_GW2_C10_0/6(R_CAN3_BMS1)
  [R_CAN3_BMS3] -> Sys_P_CAN2_GW2_C10_0/7(R_CAN3_BMS3)
  [R_CAN3_CCU1] -> Sys_P_CAN2_GW2_C10_0/8(R_CAN3_CCU1)
  [R_CAN3_EBM1] -> Sys_P_CAN2_GW2_C10_0/9(R_CAN3_EBM1)
  [R_CAN4_ZONE_DR1] -> Sys_P_CAN2_GW2_C10_0/10(R_CAN4_ZONE_DR1)
  [R_CAN4_ZONE_DR_VCU] -> Sys_P_CAN2_GW2_C10_0/11(R_CAN4_ZONE_DR_VCU)
  [R_CAN4_ZONE_FR1] -> Sys_P_CAN2_GW2_C10_0/12(R_CAN4_ZONE_FR1)
  [R_CAN4_ZONE_FR_VCU] -> Sys_P_CAN2_GW2_C10_0/13(R_CAN4_ZONE_FR_VCU)
  [R_CAN3_BMS3] -> Sys_P_CAN2_GW2_CE1000_0/1(R_CAN3_BMS3)
  [R_CAN3_MCU_B_F2] -> Sys_P_CAN2_GW2_CE1000_0/2(R_CAN3_MCU_B_F2)
  [R_CAN3_MCU_B_R2] -> Sys_P_CAN2_GW2_CE1000_0/3(R_CAN3_MCU_B_R2)
  [R_CAN3_MCU_N_F3] -> Sys_P_CAN2_GW2_CE1000_0/4(R_CAN3_MCU_N_F3)
  [R_CAN3_MCU_N_R3] -> Sys_P_CAN2_GW2_CE1000_0/5(R_CAN3_MCU_N_R3)
  [R_CAN4_PTG1] -> Sys_P_CAN2_GW2_CE1000_0/6(R_CAN4_PTG1)
  [R_CAN4_zGW_SEAT1] -> Sys_P_CAN2_GW2_CE1000_0/7(R_CAN4_zGW_SEAT1)
  [R_CAN5_TBOX3] -> Sys_P_CAN2_GW2_CE1000_0/8(R_CAN5_TBOX3)
  [R_CAN3_BMS4] -> Sys_P_CAN2_CGW_GW2_CE100_0/1(R_CAN3_BMS4)
  [R_CAN3_BMS5] -> Sys_P_CAN2_CGW_GW2_CE100_0/2(R_CAN3_BMS5)
  [R_CAN3_BMS6] -> Sys_P_CAN2_CGW_GW2_CE100_0/3(R_CAN3_BMS6)
  [R_CAN3_BMS8] -> Sys_P_CAN2_CGW_GW2_CE100_0/4(R_CAN3_BMS8)
  [R_CAN3_CCU2] -> Sys_P_CAN2_CGW_GW2_CE100_0/5(R_CAN3_CCU2)
  [R_CAN3_Shifter1] -> Sys_P_CAN2_CGW_GW2_CE100_0/6(R_CAN3_Shifter1)
  [R_CAN4_DKC1] -> Sys_P_CAN2_CGW_GW2_CE100_0/7(R_CAN4_DKC1)
  [R_CAN4_ZONE_FR1] -> Sys_P_CAN2_CGW_GW2_CE100_0/8(R_CAN4_ZONE_FR1)
  [R_CAN4_zGW_APTC1] -> Sys_P_CAN2_CGW_GW2_CE100_0/9(R_CAN4_zGW_APTC1)
  [R_CAN4_zGW_CANFr1] -> Sys_P_CAN2_CGW_GW2_CE100_0/10(R_CAN4_zGW_CANFr1)
  [R_CAN4_zGW_LINDr1] -> Sys_P_CAN2_CGW_GW2_CE100_0/11(R_CAN4_zGW_LINDr1)
  [R_CAN5_TBOX1] -> Sys_P_CAN2_CGW_GW2_CE100_0/12(R_CAN5_TBOX1)
  [R_CAN3_MCU_B_F1] -> Sys_P_CAN2_GW2_CE100_1/1(R_CAN3_MCU_B_F1)
  [R_CAN3_MCU_B_F2] -> Sys_P_CAN2_GW2_CE100_1/2(R_CAN3_MCU_B_F2)
  [R_CAN3_MCU_B_R1] -> Sys_P_CAN2_GW2_CE100_1/3(R_CAN3_MCU_B_R1)
  [R_CAN3_MCU_B_R2] -> Sys_P_CAN2_GW2_CE100_1/4(R_CAN3_MCU_B_R2)
  [R_CAN4_BodyZone_DR1] -> Sys_P_CAN2_GW2_CE100_1/5(R_CAN4_BodyZone_DR1)
  [R_CAN4_BodyZone_PS1] -> Sys_P_CAN2_GW2_CE100_1/6(R_CAN4_BodyZone_PS1)
  [R_CAN4_BodyZone_PS2] -> Sys_P_CAN2_GW2_CE100_1/7(R_CAN4_BodyZone_PS2)
  [R_CAN4_zGW_LINDr1] -> Sys_P_CAN2_GW2_CE100_1/8(R_CAN4_zGW_LINDr1)
  [R_CAN3_MCU_N_F1] -> Sys_P_CAN2_GW2_CE100_2/1(R_CAN3_MCU_N_F1)
  [R_CAN3_MCU_N_F2] -> Sys_P_CAN2_GW2_CE100_2/2(R_CAN3_MCU_N_F2)
  [R_CAN3_MCU_N_R1] -> Sys_P_CAN2_GW2_CE100_2/3(R_CAN3_MCU_N_R1)
  [R_CAN3_MCU_N_R2] -> Sys_P_CAN2_GW2_CE100_2/4(R_CAN3_MCU_N_R2)
  [R_CAN4_PTG1] -> Sys_P_CAN2_GW2_CE100_2/5(R_CAN4_PTG1)
  [R_CAN4_zGW_LINDr1] -> Sys_P_CAN2_GW2_CE100_2/6(R_CAN4_zGW_LINDr1)
  [R_CAN4_zGW_SEAT1] -> Sys_P_CAN2_GW2_CE100_2/7(R_CAN4_zGW_SEAT1)
  [R_CAN1_ESC5] -> Sys_P_CAN2_CGW_GW2_CE200_0/1(R_CAN1_ESC5)
  [R_CAN3_BMS3] -> Sys_P_CAN2_CGW_GW2_CE200_0/2(R_CAN3_BMS3)
  [R_CAN3_MCU_B_F1] -> Sys_P_CAN2_CGW_GW2_CE200_0/3(R_CAN3_MCU_B_F1)
  [R_CAN3_MCU_B_R1] -> Sys_P_CAN2_CGW_GW2_CE200_0/4(R_CAN3_MCU_B_R1)
  [R_CAN6_FCM1] -> Sys_P_CAN2_CGW_GW2_CE200_0/5(R_CAN6_FCM1)
  [R_CAN1_ABM1] -> Sys_P_CAN3_GW3_CE100_0/1(R_CAN1_ABM1)
  [R_CAN1_ESC1] -> Sys_P_CAN3_GW3_CE100_0/2(R_CAN1_ESC1)
  [R_CAN2_IVI1] -> Sys_P_CAN3_GW3_CE100_0/3(R_CAN2_IVI1)
  [R_CAN2_IVI2] -> Sys_P_CAN3_GW3_CE100_0/4(R_CAN2_IVI2)
  [R_CAN4_ZONE_FR1] -> Sys_P_CAN3_GW3_CE100_0/5(R_CAN4_ZONE_FR1)
  [R_CAN4_zGW_CANFr1] -> Sys_P_CAN3_GW3_CE100_0/6(R_CAN4_zGW_CANFr1)
  [R_CAN5_TBOX3] -> Sys_P_CAN3_GW3_CE100_0/7(R_CAN5_TBOX3)
  [R_CAN1_ESC1] -> Sys_P_CAN4_CGW_GW4_CE100_0/1(R_CAN1_ESC1)
  [R_CAN1_ESC5] -> Sys_P_CAN4_CGW_GW4_CE100_0/2(R_CAN1_ESC5)
  [R_CAN2_HMI1] -> Sys_P_CAN4_CGW_GW4_CE100_0/3(R_CAN2_HMI1)
  [R_CAN2_IVI1] -> Sys_P_CAN4_CGW_GW4_CE100_0/4(R_CAN2_IVI1)
  [R_CAN2_IVI2] -> Sys_P_CAN4_CGW_GW4_CE100_0/5(R_CAN2_IVI2)
  [R_CAN2_METER1] -> Sys_P_CAN4_CGW_GW4_CE100_0/6(R_CAN2_METER1)
  [R_CAN3_BMS6] -> Sys_P_CAN4_CGW_GW4_CE100_0/7(R_CAN3_BMS6)
  [R_CAN3_CCU2] -> Sys_P_CAN4_CGW_GW4_CE100_0/8(R_CAN3_CCU2)
  [R_CAN5_TBOX1] -> Sys_P_CAN4_CGW_GW4_CE100_0/9(R_CAN5_TBOX1)
  [R_CAN2_IVI3] -> Sys_P_CAN4_GW4_CE200_0/1(R_CAN2_IVI3)
  [R_CAN1_ABM1] -> Sys_P_CAN5_GW5_CE100_0/1(R_CAN1_ABM1)
  [R_CAN1_ESC1] -> Sys_P_CAN5_GW5_CE100_0/2(R_CAN1_ESC1)
  [R_CAN1_ESC5] -> Sys_P_CAN5_GW5_CE100_0/3(R_CAN1_ESC5)
  [R_CAN4_BodyZone_PS1] -> Sys_P_CAN5_GW5_CE100_0/4(R_CAN4_BodyZone_PS1)
  [R_CAN4_PTG1] -> Sys_P_CAN5_GW5_CE100_0/5(R_CAN4_PTG1)
  [R_CAN4_zGW_LINDr1] -> Sys_P_CAN5_GW5_CE100_0/6(R_CAN4_zGW_LINDr1)
  [R_CAN2_IVI1] -> Sys_P_CAN6_CGW_GW6_CE100_0/1(R_CAN2_IVI1)
  [R_CAN2_METER1] -> Sys_P_CAN6_CGW_GW6_CE100_0/2(R_CAN2_METER1)
  [R_CAN4_zGW_LINDr1] -> Sys_P_CAN6_CGW_GW6_CE100_0/3(R_CAN4_zGW_LINDr1)
  [R_CAN1_ESC1] -> Sys_P_CAN7_GW7_C100_0/1(R_CAN1_ESC1)

== system SWC_CGW_type/run_SWC_CGW_sys/CGW/Sys_P_CAN1_GW1_CE100_0 ==
  R_CAN3_BMS6 : Inport
  R_CAN3_MCU_B_F1 : Inport  Port=2
  R_CAN3_MCU_B_R1 : Inport  Port=3
  bus_creator : BusCreator  Inputs=3  OutDataTypeStr=Bus: DT_CAN1_SG_GW1_CE100_0  NonVirtualBus=on
  bus_selector : BusSelector  OutputSignals=CAN3_BMS_READY
  bus_selector1 : BusSelector  OutputSignals=CAN3_Fr_TMSpd
  bus_selector2 : BusSelector  OutputSignals=CAN3_Rr_TMSpd
  P_CAN1_GW1_CE100_0 : Outport
  wires:
  bus_creator/1 -> P_CAN1_GW1_CE100_0/1
  bus_selector/1 -> bus_creator/1  "<CAN3_BMS_READY>"
  [R_CAN3_BMS6] -> bus_selector/1
  bus_selector1/1 -> bus_creator/2  "<CAN3_Fr_TMSpd>"
  [R_CAN3_MCU_B_F1] -> bus_selector1/1
  bus_selector2/1 -> bus_creator/3  "<CAN3_Rr_TMSpd>"
  [R_CAN3_MCU_B_R1] -> bus_selector2/1
  R_CAN3_BMS6/1 -> [R_CAN3_BMS6]
  R_CAN3_MCU_B_F1/1 -> [R_CAN3_MCU_B_F1]
  R_CAN3_MCU_B_R1/1 -> [R_CAN3_MCU_B_R1]

== system SWC_CGW_type/run_SWC_CGW_sys/CGW/Sys_P_CAN1_GW1_CE200_0 ==
  R_CAN2_IVI2 : Inport
  bus_creator : BusCreator  Inputs=4  OutDataTypeStr=Bus: DT_CAN1_SG_GW1_CE200_0  NonVirtualBus=on
  bus_selector : BusSelector  OutputSignals=CAN2_ESC_SW_Cmd
  bus_selector1 : BusSelector  OutputSignals=CAN2_Roll_Eng_Mode
  bus_selector2 : BusSelector  OutputSignals=CAN2_Roll_Mode_SW_Cmd
  bus_selector3 : BusSelector  OutputSignals=CAN2_TCS_SW_Cmd
  P_CAN1_GW1_CE200_0 : Outport
  wires:
  bus_creator/1 -> P_CAN1_GW1_CE200_0/1
  bus_selector/1 -> bus_creator/1  "<CAN2_ESC_SW_Cmd>"
  [R_CAN2_IVI2] -> bus_selector/1
  bus_selector1/1 -> bus_creator/2  "<CAN2_Roll_Eng_Mode>"
  [R_CAN2_IVI2] -> bus_selector1/1
  bus_selector2/1 -> bus_creator/3  "<CAN2_Roll_Mode_SW_Cmd>"
  [R_CAN2_IVI2] -> bus_selector2/1
  bus_selector3/1 -> bus_creator/4  "<CAN2_TCS_SW_Cmd>"
  [R_CAN2_IVI2] -> bus_selector3/1
  R_CAN2_IVI2/1 -> [R_CAN2_IVI2]

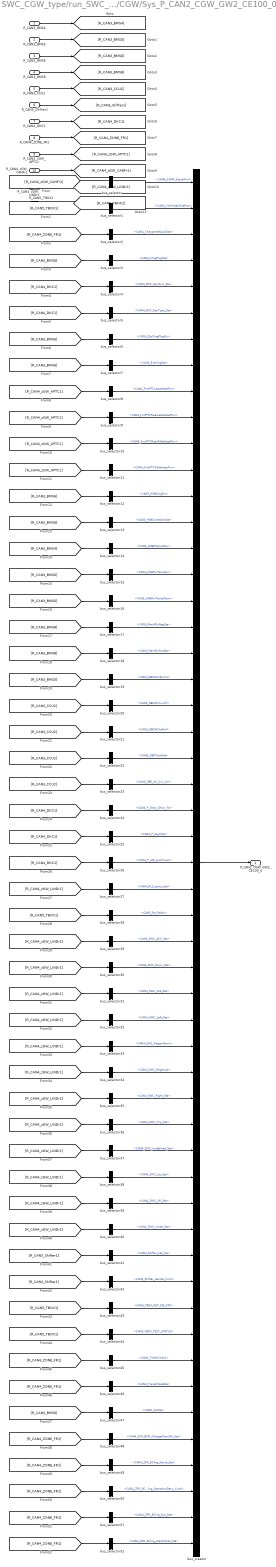
== system SWC_CGW_type/run_SWC_CGW_sys/CGW/Sys_P_CAN2_CGW_GW2_CE100_0 ==
  R_CAN3_BMS4 : Inport
  R_CAN3_BMS5 : Inport  Port=2
  R_CAN3_BMS6 : Inport  Port=3
  R_CAN3_BMS8 : Inport  Port=4
  R_CAN3_CCU2 : Inport  Port=5
  R_CAN3_Shifter1 : Inport  Port=6
  R_CAN4_DKC1 : Inport  Port=7
  R_CAN4_ZONE_FR1 : Inport  Port=8
  R_CAN4_zGW_APTC1 : Inport  Port=9
  R_CAN4_zGW_CANFr1 : Inport  Port=10
  R_CAN4_zGW_LINDr1 : Inport  Port=11
  R_CAN5_TBOX1 : Inport  Port=12
  bus_creator : BusCreator  Inputs=53  OutDataTypeStr=Bus: DT_CAN2_SG_CGW_GW2_CE100_0  NonVirtualBus=on
  bus_selector : BusSelector  OutputSignals=CAN4_COMP_ActualPwr
  bus_selector1 : BusSelector  OutputSignals=CAN5_CbnPreACEnaReq
  bus_selector10 : BusSelector  OutputSignals=CAN4_FrntPTCRearRiActHeatPwr
  bus_selector11 : BusSelector  OutputSignals=CAN4_FrntPTCRiActHeatPwr
  bus_selector12 : BusSelector  OutputSignals=CAN3_HVBChrgErr
  bus_selector13 : BusSelector  OutputSignals=CAN3_HVBContactorSta
  bus_selector14 : BusSelector  OutputSignals=CAN3_HVBMTempMax
  bus_selector15 : BusSelector  OutputSignals=CAN3_HVBOvrTempErr
  bus_selector16 : BusSelector  OutputSignals=CAN3_HVBOvrTempWarn
  bus_selector17 : BusSelector  OutputSignals=CAN3_MainRlyNegSta
  bus_selector18 : BusSelector  OutputSignals=CAN3_MainRlyPosSta
  bus_selector19 : BusSelector  OutputSignals=CAN3_OBCACCSLimit
  bus_selector2 : BusSelector  OutputSignals=CAN4_ChargeInletLockSta
  bus_selector20 : BusSelector  OutputSignals=CAN3_OBCACCurrInf
  bus_selector21 : BusSelector  OutputSignals=CAN3_OBCACVoltInf
  bus_selector22 : BusSelector  OutputSignals=CAN3_OBCFaultSta
  bus_selector23 : BusSelector  OutputSignals=CAN3_OBC_AC_Cur_Lim
  bus_selector24 : BusSelector  OutputSignals=CAN4_P_Dkey_Show_IVI
  bus_selector25 : BusSelector  OutputSignals=CAN4_P_KeyMiss
  bus_selector26 : BusSelector  OutputSignals=CAN4_P_UID_LowPower
  bus_selector27 : BusSelector  OutputSignals=CAN4_RLS_Lamp_Sta
  bus_selector28 : BusSelector  OutputSignals=CAN5_Re_Radio
  bus_selector29 : BusSelector  OutputSignals=CAN4_SWC_ACC_Sta
  bus_selector3 : BusSelector  OutputSignals=CAN3_ChrgPlugSta
  bus_selector30 : BusSelector  OutputSignals=CAN4_SWC_Down_Sta
  bus_selector31 : BusSelector  OutputSignals=CAN4_SWC_LKA_Sta
  bus_selector32 : BusSelector  OutputSignals=CAN4_SWC_Left_Sta
  bus_selector33 : BusSelector  OutputSignals=CAN4_SWC_RegenDown
  bus_selector34 : BusSelector  OutputSignals=CAN4_SWC_RegenUp
  bus_selector35 : BusSelector  OutputSignals=CAN4_SWC_Right_Sta
  bus_selector36 : BusSelector  OutputSignals=CAN4_SWC_Trip_Sta
  bus_selector37 : BusSelector  OutputSignals=CAN4_SWC_Undefined_Sta
  bus_selector38 : BusSelector  OutputSignals=CAN4_SWC_Up_Sta
  bus_selector39 : BusSelector  OutputSignals=CAN4_SWC_VR_Sta
  bus_selector4 : BusSelector  OutputSignals=CAN4_DKC_KeyNum_Sta
  bus_selector40 : BusSelector  OutputSignals=CAN4_SWC_mode_Sta
  bus_selector41 : BusSelector  OutputSignals=CAN3_Shifter_Fail_sta
  bus_selector42 : BusSelector  OutputSignals=CAN3_Shifter_Handle_Cmd
  bus_selector43 : BusSelector  OutputSignals=CAN5_TBOX_NET_SIG_STR
  bus_selector44 : BusSelector  OutputSignals=CAN5_TBOX_TEST_STATUS
  bus_selector45 : BusSelector  OutputSignals=CAN4_TrailerCheck
  bus_selector46 : BusSelector  OutputSignals=CAN4_TrailerModeSta
  bus_selector47 : BusSelector  OutputSignals=CAN3_V2LSta
  bus_selector48 : BusSelector  OutputSignals=CAN4_ZFR_BCM_ChargerDoorSW_Sta
  bus_selector49 : BusSelector  OutputSignals=CAN4_ZFR_EChrg_Active_Sta
  bus_selector5 : BusSelector  OutputSignals=CAN4_DKC_KeyType_Sta
  bus_selector50 : BusSelector  OutputSignals=CAN4_ZFR_EChrg_OperationDeny_Cmd
  bus_selector51 : BusSelector  OutputSignals=CAN4_ZFR_EChrg_Sys_Sta
  bus_selector52 : BusSelector  OutputSignals=CAN4_ZFR_EChrg_WashMode_Sta
  bus_selector6 : BusSelector  OutputSignals=CAN3_DisChrgPlugErr
  bus_selector7 : BusSelector  OutputSignals=CAN3_ExtChrgSta
  bus_selector8 : BusSelector  OutputSignals=CAN4_FrntPTCLeActHeatPwr
  bus_selector9 : BusSelector  OutputSignals=CAN4_FrntPTCRearLeActHeatPwr
  P_CAN2_CGW_GW2_CE100_0 : Outport
  wires:
  bus_creator/1 -> P_CAN2_CGW_GW2_CE100_0/1
  bus_selector/1 -> bus_creator/1  "<CAN4_COMP_ActualPwr>"
  [R_CAN4_zGW_CANFr1] -> bus_selector/1
  bus_selector1/1 -> bus_creator/2  "<CAN5_CbnPreACEnaReq>"
  [R_CAN5_TBOX1] -> bus_selector1/1
  bus_selector2/1 -> bus_creator/3  "<CAN4_ChargeInletLockSta>"
  [R_CAN4_ZONE_FR1] -> bus_selector2/1
  bus_selector3/1 -> bus_creator/4  "<CAN3_ChrgPlugSta>"
  [R_CAN3_BMS6] -> bus_selector3/1
  bus_selector4/1 -> bus_creator/5  "<CAN4_DKC_KeyNum_Sta>"
  [R_CAN4_DKC1] -> bus_selector4/1
  bus_selector5/1 -> bus_creator/6  "<CAN4_DKC_KeyType_Sta>"
  [R_CAN4_DKC1] -> bus_selector5/1
  bus_selector6/1 -> bus_creator/7  "<CAN3_DisChrgPlugErr>"
  [R_CAN3_BMS6] -> bus_selector6/1
  bus_selector7/1 -> bus_creator/8  "<CAN3_ExtChrgSta>"
  [R_CAN3_BMS6] -> bus_selector7/1
  bus_selector8/1 -> bus_creator/9  "<CAN4_FrntPTCLeActHeatPwr>"
  [R_CAN4_zGW_APTC1] -> bus_selector8/1
  bus_selector9/1 -> bus_creator/10  "<CAN4_FrntPTCRearLeActHeatPwr>"
  [R_CAN4_zGW_APTC1] -> bus_selector9/1
  bus_selector10/1 -> bus_creator/11  "<CAN4_FrntPTCRearRiActHeatPwr>"
  [R_CAN4_zGW_APTC1] -> bus_selector10/1
  bus_selector11/1 -> bus_creator/12  "<CAN4_FrntPTCRiActHeatPwr>"
  [R_CAN4_zGW_APTC1] -> bus_selector11/1
  bus_selector12/1 -> bus_creator/13  "<CAN3_HVBChrgErr>"
  [R_CAN3_BMS6] -> bus_selector12/1
  bus_selector13/1 -> bus_creator/14  "<CAN3_HVBContactorSta>"
  [R_CAN3_BMS6] -> bus_selector13/1
  bus_selector14/1 -> bus_creator/15  "<CAN3_HVBMTempMax>"
  [R_CAN3_BMS4] -> bus_selector14/1
  bus_selector15/1 -> bus_creator/16  "<CAN3_HVBOvrTempErr>"
  [R_CAN3_BMS6] -> bus_selector15/1
  bus_selector16/1 -> bus_creator/17  "<CAN3_HVBOvrTempWarn>"
  [R_CAN3_BMS6] -> bus_selector16/1
  bus_selector17/1 -> bus_creator/18  "<CAN3_MainRlyNegSta>"
  [R_CAN3_BMS8] -> bus_selector17/1
  bus_selector18/1 -> bus_creator/19  "<CAN3_MainRlyPosSta>"
  [R_CAN3_BMS8] -> bus_selector18/1
  bus_selector19/1 -> bus_creator/20  "<CAN3_OBCACCSLimit>"
  [R_CAN3_BMS5] -> bus_selector19/1
  bus_selector20/1 -> bus_creator/21  "<CAN3_OBCACCurrInf>"
  [R_CAN3_CCU2] -> bus_selector20/1
  bus_selector21/1 -> bus_creator/22  "<CAN3_OBCACVoltInf>"
  [R_CAN3_CCU2] -> bus_selector21/1
  bus_selector22/1 -> bus_creator/23  "<CAN3_OBCFaultSta>"
  [R_CAN3_CCU2] -> bus_selector22/1
  bus_selector23/1 -> bus_creator/24  "<CAN3_OBC_AC_Cur_Lim>"
  [R_CAN3_CCU2] -> bus_selector23/1
  bus_selector24/1 -> bus_creator/25  "<CAN4_P_Dkey_Show_IVI>"
  [R_CAN4_DKC1] -> bus_selector24/1
  bus_selector25/1 -> bus_creator/26  "<CAN4_P_KeyMiss>"
  [R_CAN4_DKC1] -> bus_selector25/1
  bus_selector26/1 -> bus_creator/27  "<CAN4_P_UID_LowPower>"
  [R_CAN4_DKC1] -> bus_selector26/1
  bus_selector27/1 -> bus_creator/28  "<CAN4_RLS_Lamp_Sta>"
  [R_CAN4_zGW_LINDr1] -> bus_selector27/1
  bus_selector28/1 -> bus_creator/29  "<CAN5_Re_Radio>"
  [R_CAN5_TBOX1] -> bus_selector28/1
  bus_selector29/1 -> bus_creator/30  "<CAN4_SWC_ACC_Sta>"
  [R_CAN4_zGW_LINDr1] -> bus_selector29/1
  bus_selector30/1 -> bus_creator/31  "<CAN4_SWC_Down_Sta>"
  [R_CAN4_zGW_LINDr1] -> bus_selector30/1
  bus_selector31/1 -> bus_creator/32  "<CAN4_SWC_LKA_Sta>"
  [R_CAN4_zGW_LINDr1] -> bus_selector31/1
  bus_selector32/1 -> bus_creator/33  "<CAN4_SWC_Left_Sta>"
  [R_CAN4_zGW_LINDr1] -> bus_selector32/1
  bus_selector33/1 -> bus_creator/34  "<CAN4_SWC_RegenDown>"
  [R_CAN4_zGW_LINDr1] -> bus_selector33/1
  bus_selector34/1 -> bus_creator/35  "<CAN4_SWC_RegenUp>"
  [R_CAN4_zGW_LINDr1] -> bus_selector34/1
  bus_selector35/1 -> bus_creator/36  "<CAN4_SWC_Right_Sta>"
  [R_CAN4_zGW_LINDr1] -> bus_selector35/1
  bus_selector36/1 -> bus_creator/37  "<CAN4_SWC_Trip_Sta>"
  [R_CAN4_zGW_LINDr1] -> bus_selector36/1
  bus_selector37/1 -> bus_creator/38  "<CAN4_SWC_Undefined_Sta>"
  [R_CAN4_zGW_LINDr1] -> bus_selector37/1
  bus_selector38/1 -> bus_creator/39  "<CAN4_SWC_Up_Sta>"
  [R_CAN4_zGW_LINDr1] -> bus_selector38/1
  bus_selector39/1 -> bus_creator/40  "<CAN4_SWC_VR_Sta>"
  [R_CAN4_zGW_LINDr1] -> bus_selector39/1
  bus_selector40/1 -> bus_creator/41  "<CAN4_SWC_mode_Sta>"
  [R_CAN4_zGW_LINDr1] -> bus_selector40/1
  bus_selector41/1 -> bus_creator/42  "<CAN3_Shifter_Fail_sta>"
  [R_CAN3_Shifter1] -> bus_selector41/1
  bus_selector42/1 -> bus_creator/43  "<CAN3_Shifter_Handle_Cmd>"
  [R_CAN3_Shifter1] -> bus_selector42/1
  bus_selector43/1 -> bus_creator/44  "<CAN5_TBOX_NET_SIG_STR>"
  [R_CAN5_TBOX1] -> bus_selector43/1
  bus_selector44/1 -> bus_creator/45  "<CAN5_TBOX_TEST_STATUS>"
  [R_CAN5_TBOX1] -> bus_selector44/1
  bus_selector45/1 -> bus_creator/46  "<CAN4_TrailerCheck>"
  [R_CAN4_ZONE_FR1] -> bus_selector45/1
  bus_selector46/1 -> bus_creator/47  "<CAN4_TrailerModeSta>"
  [R_CAN4_ZONE_FR1] -> bus_selector46/1
  bus_selector47/1 -> bus_creator/48  "<CAN3_V2LSta>"
  [R_CAN3_BMS6] -> bus_selector47/1
  bus_selector48/1 -> bus_creator/49  "<CAN4_ZFR_BCM_ChargerDoorSW_Sta>"
  [R_CAN4_ZONE_FR1] -> bus_selector48/1
  bus_selector49/1 -> bus_creator/50  "<CAN4_ZFR_EChrg_Active_Sta>"
  [R_CAN4_ZONE_FR1] -> bus_selector49/1
  bus_selector50/1 -> bus_creator/51  "<CAN4_ZFR_EChrg_OperationDeny_Cmd>"
  [R_CAN4_ZONE_FR1] -> bus_selector50/1
  bus_selector51/1 -> bus_creator/52  "<CAN4_ZFR_EChrg_Sys_Sta>"
  [R_CAN4_ZONE_FR1] -> bus_selector51/1
  bus_selector52/1 -> bus_creator/53  "<CAN4_ZFR_EChrg_WashMode_Sta>"
  [R_CAN4_ZONE_FR1] -> bus_selector52/1
  R_CAN3_BMS4/1 -> [R_CAN3_BMS4]
  R_CAN3_BMS5/1 -> [R_CAN3_BMS5]
  R_CAN3_BMS6/1 -> [R_CAN3_BMS6]
  R_CAN3_BMS8/1 -> [R_CAN3_BMS8]
  R_CAN3_CCU2/1 -> [R_CAN3_CCU2]
  R_CAN3_Shifter1/1 -> [R_CAN3_Shifter1]
  R_CAN4_DKC1/1 -> [R_CAN4_DKC1]
  R_CAN4_ZONE_FR1/1 -> [R_CAN4_ZONE_FR1]
  R_CAN4_zGW_APTC1/1 -> [R_CAN4_zGW_APTC1]
  R_CAN4_zGW_CANFr1/1 -> [R_CAN4_zGW_CANFr1]
  R_CAN4_zGW_LINDr1/1 -> [R_CAN4_zGW_LINDr1]
  R_CAN5_TBOX1/1 -> [R_CAN5_TBOX1]
